simulink model "misc"  (R2025a)
settings: Solver=VariableStepAuto  StartTime=0.0  StopTime=10.0  RelTol=1e-3
undefined symbols (not defined in the file): Acid, Lead
libraries: spsBatteryLib x1, spsGroundLib x1, spspowerguiLib x1
settings Model: Creator=GNKRISHNAN  LastModifiedBy=GNKRISHNAN

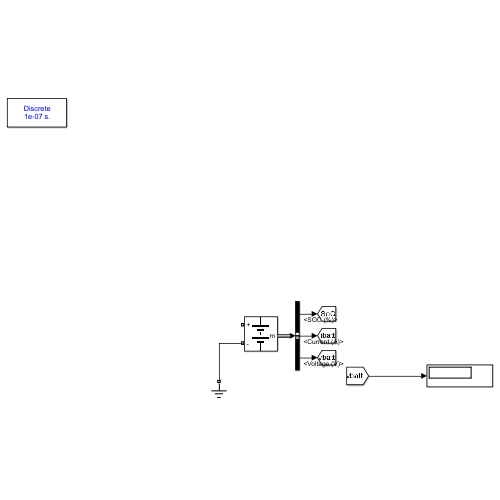
[thumbnail: Simulink's stored preview of the top-level diagram]
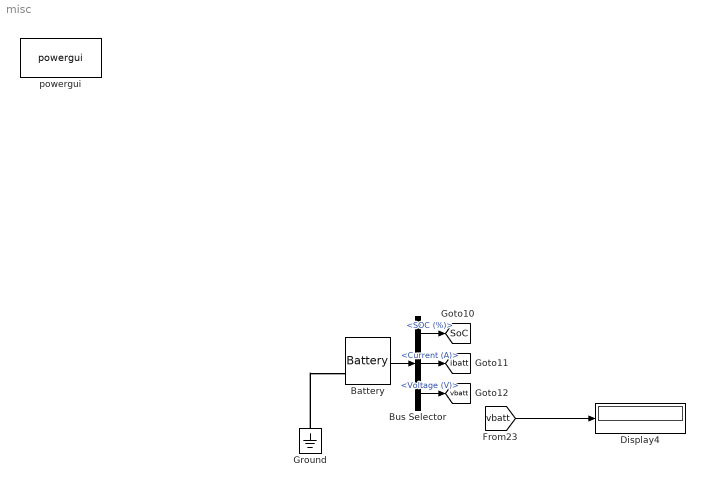
== system misc ==
  Battery : spsBatteryLib/Battery  BatType=Lead-Acid  NomV=12  NomQ=6.4  SOC=90  Batt_Tr=1  PresetModel=on  MaxQ=6.6667  MinV=9  FullV=13.0658  Dis_rate=1.28  R=0.01875  Normal_OP=1.9858  expZone="[12.2171    0.0213333]"
  Bus Selector : BusSelector  OutputSignals=SOC (%),Current (A),Voltage (V)
  Display4 : Display
  Ground : spsGroundLib/Ground  LConnTagsString=a
  powergui : spspowerguiLib/powergui  Priority=1  SimulationMode=Discrete  SampleTime=1e-7  frequency=60  Iterations=50  frequencyindice=0  Pbase=100e6  ErrMax=1e-4  UnitsV=kV  UnitsW=MW  buscounter=0  FunctionMessages=off  echomessages=off  EnableUseOfTLC=off  CurrentSourceSwitches=off  DisableSnubberDevices=off  DisableRonSwitches=off  DisableVfSwitches=off  DisplayEquations=off  AutomaticDiscreteSolvers=off  SolverType=Tustin/Backward Euler (TBE)  Interpol=off  ExternalGateDelay=off  methode=off  Ts=100  x0status=blocks  SPID=on  SwTol=0  HookPort=off  NonlinearTolerance=1e-4  nMaxIteration=100  ContinueOnMaxIteration=off  RestoreLinks=warning  ResistiveCurrentMeasurement=off  Frange=[0:2:500]  Ylog=off  Xlog=on  ShowGrid=off  save=off  variable=ZData  structure=0  ZoomFFT=off  StartTime=0.0  cycles=1  DisplayStyle=1  fundamental=60  FreqAxis=off  MaxFrequency=1000  frequencyindicesteady=1  RmsSteady=1  display=off
  tag scope: SoC=global, ibatt=global, vbatt=global
  wires:
  Bus Selector/2 -> [ibatt]  "<Current (A)>"
  Battery/1 -> Bus Selector/1
  Bus Selector/1 -> [SoC]  "<SOC (%)>"
  Bus Selector/3 -> [vbatt]  "<Voltage (V)>"
  [vbatt] -> Display4/1
  connections:
  Ground/LConn1 -- Battery/LConn2
